simulink model "ModellVerifikation"  (R2015b)
settings: Solver=ode1  StartTime=0.0  StopTime=Tend  FixedStep=Tstep  RelTol=1e-3
PreLoadFcn:
  | run ModellInit
  | Tstep = 0.001;
settings Model: Creator=Amann  LastModifiedBy=Amann
settings DataIOCC: SaveFormat=Array
settings DebuggingCC: UnderspecifiedInitializationDetection=Classic  MergeDetectMultiDrivingBlocksExec=none  SolverPrmCheckMsg=warning  StateNameClashWarn=warning
settings HardwareCC: ProdBitPerPointer=32  ProdLargestAtomicFloat=None  ProdIntDivRoundTo=Undefined  ProdEndianess=Unspecified  ProdWordSize=32  ProdHWDeviceType=32-bit Generic
settings GRTTargetCC: GeneratePreprocessorConditionals=Disable all
settings ConfigComp: CovModelRefEnable=Off

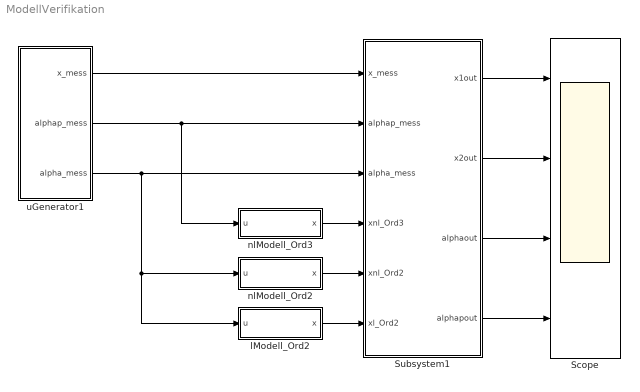
== system ModellVerifikation ==
  Scope : Scope  NumInputPorts=4
  Subsystem1 : Subsystem
  lModell_Ord2 : Subsystem
  nlModell_Ord2 : Subsystem
  nlModell_Ord3 : Subsystem
  uGenerator1 : Subsystem
  wires:
  nlModell_Ord3/1(x) -> Subsystem1/4(xnl_Ord3)
  Subsystem1/1(x1out) -> Scope/1
  Subsystem1/2(x2out) -> Scope/2
  Subsystem1/3(alphaout) -> Scope/3
  Subsystem1/4(alphapout) -> Scope/4
  uGenerator1/2(alphap_mess) -> Subsystem1/2(alphap_mess), nlModell_Ord3/1(u)
  uGenerator1/1(x_mess) -> Subsystem1/1(x_mess)
  uGenerator1/3(alpha_mess) -> Subsystem1/3(alpha_mess), lModell_Ord2/1(u), nlModell_Ord2/1(u)
  nlModell_Ord2/1(x) -> Subsystem1/5(xnl_Ord2)
  lModell_Ord2/1(x) -> Subsystem1/6(xl_Ord2)

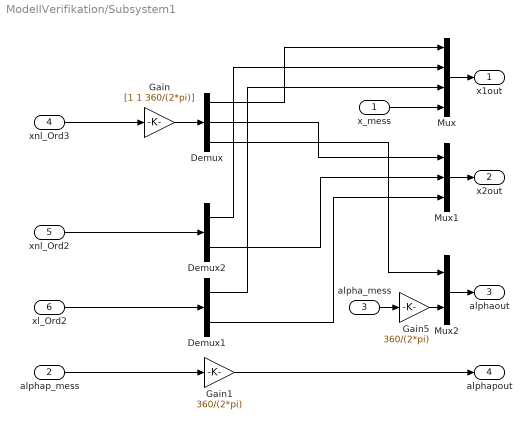
== system ModellVerifikation/Subsystem1 ==
  x_mess : Inport
  alphap_mess : Inport  Port=2
  alpha_mess : Inport  Port=3
  xnl_Ord3 : Inport  Port=4
  xnl_Ord2 : Inport  Port=5
  xl_Ord2 : Inport  Port=6
  Demux : Demux  Outputs=3
  Demux1 : Demux  Outputs=2
  Demux2 : Demux  Outputs=2
  Gain : Gain  Gain=[1 1 360/(2*pi)]
  Gain1 : Gain  Gain=360/(2*pi)
  Gain5 : Gain  Gain=360/(2*pi)
  Mux : Mux
  Mux1 : Mux  Inputs=3
  Mux2 : Mux  Inputs=2
  x1out : Outport
  x2out : Outport  Port=2
  alphaout : Outport  Port=3
  alphapout : Outport  Port=4
  wires:
  xnl_Ord3/1 -> Gain/1
  alphap_mess/1 -> Gain1/1
  Gain/1 -> Demux/1
  xl_Ord2/1 -> Demux1/1
  Mux/1 -> x1out/1
  Mux1/1 -> x2out/1
  Mux2/1 -> alphaout/1
  Demux/1 -> Mux/1
  Demux/2 -> Mux1/1
  Demux/3 -> Mux2/1
  Demux2/1 -> Mux/2
  Demux2/2 -> Mux1/2
  x_mess/1 -> Mux/4
  xnl_Ord2/1 -> Demux2/1
  Demux1/1 -> Mux/3
  Demux1/2 -> Mux1/3
  alpha_mess/1 -> Gain5/1
  Gain1/1 -> alphapout/1
  Gain5/1 -> Mux2/2

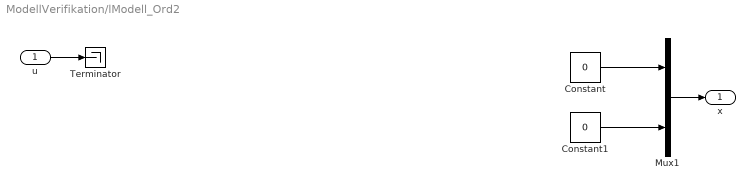
== system ModellVerifikation/lModell_Ord2 ==
  u : Inport
  Constant : Constant  Value=0
  Constant1 : Constant  Value=0
  Mux1 : Mux  Inputs=2
  Terminator : Terminator
  x : Outport
  wires:
  Mux1/1 -> x/1
  u/1 -> Terminator/1
  Constant1/1 -> Mux1/2
  Constant/1 -> Mux1/1

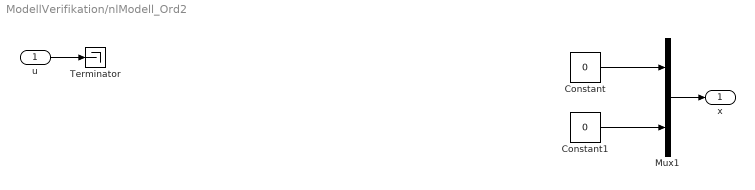
== system ModellVerifikation/nlModell_Ord2 ==
  u : Inport
  Constant : Constant  Value=0
  Constant1 : Constant  Value=0
  Mux1 : Mux  Inputs=2
  Terminator : Terminator
  x : Outport
  wires:
  Mux1/1 -> x/1
  u/1 -> Terminator/1
  Constant1/1 -> Mux1/2
  Constant/1 -> Mux1/1

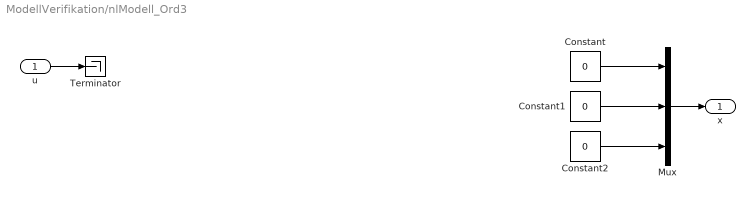
== system ModellVerifikation/nlModell_Ord3 ==
  u : Inport
  Constant : Constant  Value=0
  Constant1 : Constant  Value=0
  Constant2 : Constant  Value=0
  Mux : Mux  Inputs=3
  Terminator : Terminator
  x : Outport
  wires:
  Mux/1 -> x/1
  u/1 -> Terminator/1
  Constant1/1 -> Mux/2
  Constant2/1 -> Mux/3
  Constant/1 -> Mux/1

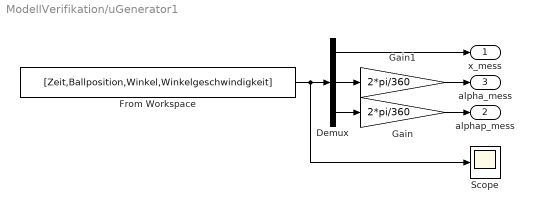
== system ModellVerifikation/uGenerator1 ==
  Demux : Demux  Outputs=3
  From Workspace : FromWorkspace  VariableName=[Zeit,Ballposition,Winkel,Winkelgeschwindigkeit]  SampleTime=0
  Gain : Gain  Gain=2*pi/360
  Gain1 : Gain  Gain=2*pi/360
  Scope : Scope
  x_mess : Outport
  alphap_mess : Outport  Port=2
  alpha_mess : Outport  Port=3
  wires:
  From Workspace/1 -> Scope/1, Demux/1
  Demux/1 -> x_mess/1
  Gain/1 -> alphap_mess/1
  Demux/3 -> Gain/1
  Demux/2 -> Gain1/1
  Gain1/1 -> alpha_mess/1
